simulink model "Blink"  (R2019b)
settings: Solver=VariableStepAuto  StartTime=0.0  StopTime=10.0  RelTol=1e-3
libraries: frdmk64flib x1
settings Model: Creator=shahv10  LastModifiedBy=shahv10

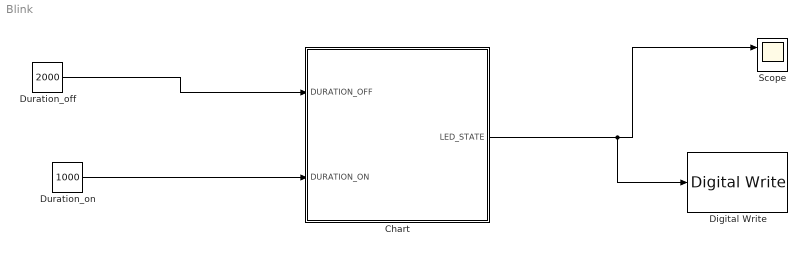
== system Blink ==
  Chart : Stateflow chart  BlockKeywords=__PRM__SERIALIZED__DATA__:Stateflow Chart,Stateflow Diagram  TreatAsAtomicUnit=on
  Digital Write : frdmk64flib/Digital Write  Whichpin=RED_LED
      settings: SourceProductName=Simulink Coder Support Package for NXP FRDM-K64F Board
  Duration_off : Constant  Value=2000  OutDataTypeStr=int16
  Duration_on : Constant  Value=1000  OutDataTypeStr=int16
  Scope : Scope  NumInputPorts=2
  wires:
  Chart/1(LED_STATE) -> Digital Write/1, Scope/1
  Duration_on/1 -> Chart/2(DURATION_ON)
  Duration_off/1 -> Chart/1(DURATION_OFF)

== stateflow chart Blink/Chart ==
  state LED_OFF
    entry:
    LED_STATE=true;
  state LED_ON
    entry:
    LED_STATE=false;
  (default) -> LED_OFF
  LED_OFF -> LED_ON : after(DURATION_OFF,msec)
  LED_ON -> LED_OFF : after(DURATION_ON,msec)
  data: LED_STATE output; DURATION_OFF input; DURATION_ON input
